simulink model "open_loop"  (R2018b)
settings: Solver=VariableStepAuto  StartTime=0.0  StopTime=100  RelTol=1e-3
undefined symbols (not defined in the file): Ax, Ay, Ayaw, Az, Bx, By, Byaw, Bz, Cx, Cy, Cyaw, Cz, Dx, Dy, Dyaw, Dz, x0x, x0y, x0yaw, x0z
settings Model: Creator=Rafik  LastModifiedBy=Rafik

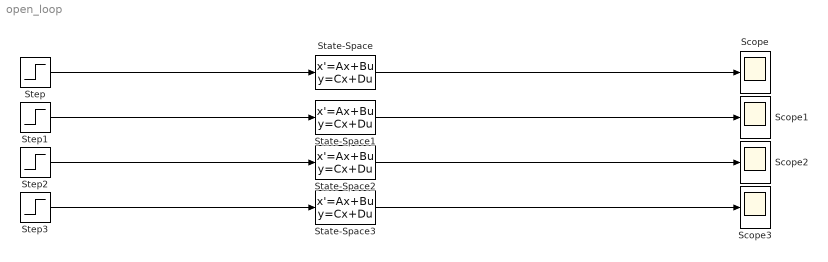
== system open_loop ==
  Scope{,1..3} (4 alike) : Scope
  State-Space : StateSpace  A=Ax  B=Bx  C=Cx  D=Dx  InitialCondition=x0x
  State-Space1 : StateSpace  A=Ay  B=By  C=Cy  D=Dy  InitialCondition=x0y
  State-Space2 : StateSpace  A=Az  B=Bz  C=Cz  D=Dz  InitialCondition=x0z
  State-Space3 : StateSpace  A=Ayaw  B=Byaw  C=Cyaw  D=Dyaw  InitialCondition=x0yaw
  Step{,1..3} (4 alike) : Step  SampleTime=0
  wires:
  State-Space/1 -> Scope/1
  State-Space2/1 -> Scope2/1
  State-Space1/1 -> Scope1/1
  Step3/1 -> State-Space3/1
  Step1/1 -> State-Space1/1
  Step2/1 -> State-Space2/1
  Step/1 -> State-Space/1
  State-Space3/1 -> Scope3/1
